simulink model "SM_Computing_Torque"  (R2015a)
settings: Solver=ode45  StartTime=0.0  StopTime=10.0  RelTol=1e-3
values from neighbouring files (symbols this model uses):
  ddq = diff([zeros(1,n); dq])./diff(tm)    [PF_Parametrised_J_ti_Traj.m]    (also in PF_Parametrised_cav_Traj.m; PF_Parametrised_ti_Traj.m; PF_Table_ti_Traj.m; SF_Dynamic_Simulation.m)
  dq = diff([zeros(1,n); q])./diff(tm)    [PF_Parametrised_J_ti_Traj.m]    (also in PF_Parametrised_cav_Traj.m = zeros(sp, n); PF_Parametrised_ti_Traj.m; PF_Table_ti_Traj.m; SF_Dynamic_Simulation.m = rad2deg(dq))
  q = H(cn - 1).q(end,:)    [MF_Plot_CG_frames.m]    (also in PF_Collision_Check.m = varargin{i+1}; PF_Conf_Const_Reach.m = varargin{i+1}; PF_Parametrised_J_ti_Traj.m = (q0' * ones(1, sp))'; PF_Parametrised_cav_Traj.m = (q0' * ones(1, sp))')
  q0 = S.value{'home_q'}    [MF_Init_Graph_Rep.m]    (also in PF_Parametrised_J_ti_Traj.m = H(cn - 1).q(end,:); PF_Parametrised_cav_Traj.m = H(cn - 1).q(end,:); PF_Parametrised_ti_Traj.m = H(cn - 1).q(end,:); PF_Table_ti_Traj.m = H(cn - 1).q(end,:))
undefined symbols (not defined in the file or in its folder): PF_Inverse_DynamicsII
settings Model: Creator=Diego  LastModifiedBy=Diego

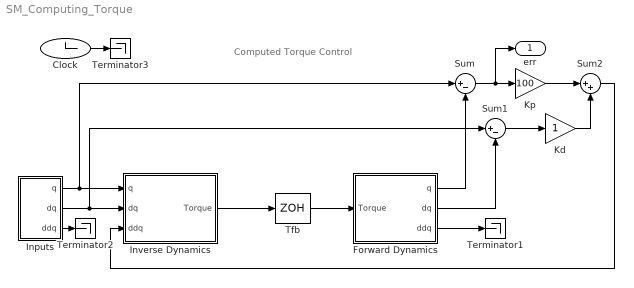
== system SM_Computing_Torque ==
  note: Computed Torque Control
  Clock : Clock
  Forward Dynamics : Subsystem
  Inputs : Subsystem
  Inverse Dynamics : Subsystem
  Kd : Gain  SaturateOnIntegerOverflow=on  OutDataTypeStr=Inherit: Same as input  ParamDataTypeStr=Inherit: Same as input
  Kp : Gain  Gain=100  SaturateOnIntegerOverflow=on  OutDataTypeStr=Inherit: Same as input  ParamDataTypeStr=Inherit: Same as input
  Sum : Sum  Inputs=|+-  SaturateOnIntegerOverflow=on  InputSameDT=on  OutDataTypeStr=Inherit: Same as first input
  Sum1 : Sum  Inputs=|+-  SaturateOnIntegerOverflow=on  InputSameDT=on  OutDataTypeStr=Inherit: Same as first input
  Sum2 : Sum  Inputs=|++  SaturateOnIntegerOverflow=on  InputSameDT=on  OutDataTypeStr=Inherit: Same as first input
  Terminator1 : Terminator
  Terminator2 : Terminator
  Terminator3 : Terminator
  Tfb : ZeroOrderHold  SampleTime=0.01
  err : Outport
  wires:
  Inputs/1(q) -> Sum/1, Inverse Dynamics/1(q)
  Inputs/2(dq) -> Sum1/1, Inverse Dynamics/2(dq)
  Inverse Dynamics/1(Torque) -> Tfb/1
  Tfb/1 -> Forward Dynamics/1(Torque)
  Forward Dynamics/3(ddq) -> Terminator1/1
  Sum/1 -> Kp/1, err/1
  Kp/1 -> Sum2/1
  Sum1/1 -> Kd/1
  Kd/1 -> Sum2/2
  Inputs/3(ddq) -> Terminator2/1
  Sum2/1 -> Inverse Dynamics/3(ddq)
  Forward Dynamics/2(dq) -> Sum1/2
  Forward Dynamics/1(q) -> Sum/2
  Clock/1 -> Terminator3/1

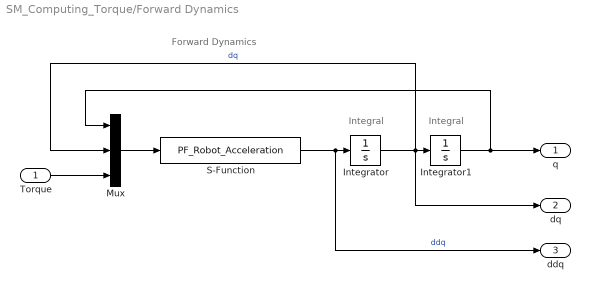
== system SM_Computing_Torque/Forward Dynamics ==
  note: Forward Dynamics
  note: Integral
  note: Integral
  Torque : Inport
  Integrator : Integrator
  Integrator1 : Integrator  InitialCondition=q0
  Mux : Mux  Inputs=3
  S-Function : S-Function  FunctionName=PF_Robot_Acceleration  Parameters=robot
  q : Outport
  dq : Outport  Port=2
  ddq : Outport  Port=3
  wires:
  Torque/1 -> Mux/3
  Mux/1 -> S-Function/1
  S-Function/1 -> ddq/1, Integrator/1  "ddq"
  Integrator/1 -> dq/1, Integrator1/1, Mux/2  "dq"
  Integrator1/1 -> q/1, Mux/1

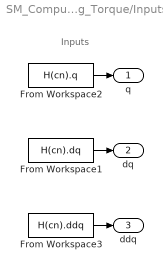
== system SM_Computing_Torque/Inputs ==
  note: Inputs
  From Workspace1 : FromWorkspace  VariableName=H(cn).dq  SampleTime=0.1
  From Workspace2 : FromWorkspace  VariableName=H(cn).q  SampleTime=0.1
  From Workspace3 : FromWorkspace  VariableName=H(cn).ddq  SampleTime=0.1
  q : Outport
  dq : Outport  Port=2
  ddq : Outport  Port=3
  wires:
  From Workspace1/1 -> dq/1
  From Workspace3/1 -> ddq/1
  From Workspace2/1 -> q/1

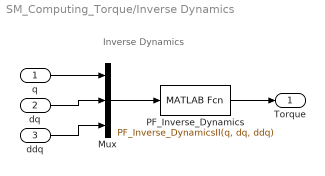
== system SM_Computing_Torque/Inverse Dynamics ==
  note: Inverse Dynamics
  q : Inport
  dq : Inport  Port=2
  ddq : Inport  Port=3
  Mux : Mux  Inputs=3
  PF_Inverse_Dynamics : MATLABFcn  MATLABFcn=PF_Inverse_DynamicsII(q, dq, ddq)  OutputDimensions=n
  Torque : Outport
  wires:
  PF_Inverse_Dynamics/1 -> Torque/1
  Mux/1 -> PF_Inverse_Dynamics/1
  q/1 -> Mux/1
  dq/1 -> Mux/2
  ddq/1 -> Mux/3
